simulink model "parallel_RFPSC_PSC_simulation"  (R2023b)
settings: Solver=VariableStepAuto  StartTime=0  StopTime=.1  FixedStep=T_s  MaxStep=T_s  RelTol=1e-4  AbsTol=1e-4  EnableMultiTasking=on
values from neighbouring files (symbols this model uses):
  f_sw = 10e3    (= 10000)    [init_psc_parallel.m]
  K_p = 3*w_g*R_a/(2*u_gN^2)    (= 0.261799387799)    [init_psc_parallel.m]
  L_f1 = L_f    (= 0.001)    [init_psc_parallel.m]
  L_f2 = L_f    (= 0.001)    [init_psc_parallel.m]
  L_g = 2.5e-3    (= 0.0025)    [init_psc_parallel.m]
  R_a = 0.32    [init_psc_parallel.m]
  R_L = 10    [init_psc_parallel.m]
  T_s = 1/(2*f_sw)    (= 5e-05)    [init_psc_parallel.m]
  U_dc = 48    [init_psc_parallel.m]
  u_gN = 24    [init_psc_parallel.m]
  w_g = 2*pi*50    (= 314.159265359)    [init_psc_parallel.m]    (also in psc_matlab.m = (P_ref - P)*K_p + w_1)
libraries: simulink x2
settings Model: Creator=mhinkkan  LastModifiedBy=jonwe
settings SolverCC: AutoScaleAbsTol=off  MaxConsecutiveMinStep=10  AlgebraicLoopSolver=TrustRegion
settings DataIOCC: SaveFormat=Array  SignalLoggingSaveFormat=ModelDataLogs  SaveOutput=off  SignalLogging=off  DSMLogging=off  SaveTime=off  ReturnWorkspaceOutputs=off
settings OptimizationCC: BlockReduction=off  BooleanDataType=off  DefaultParameterBehavior=Inlined  OptimizeBlockIOStorage=off  BufferReuse=off  ReuseModelBlockBuffer=off  ExpressionFolding=off  ExpressionDepthLimit=2147483647  LocalBlockOutputs=off  InitFltsAndDblsToZero=on  LifeSpan=inf
settings DebuggingCC: AlgebraicLoopMsg=none  SaveWithParameterizedLinksMsg=none  UnderspecifiedInitializationDetection=Classic  MergeDetectMultiDrivingBlocksExec=none  SignalResolutionControl=TryResolveAllWithWarning  MultiTaskDSMMsg=warning  MultiTaskCondExecSysMsg=none  FcnCallInpInsideContextMsg=warning  UnconnectedInputMsg=warning  UnconnectedOutputMsg=warning  UnconnectedLineMsg=warning  StateNameClashWarn=warning  SFUnexpectedBacktrackingDiag=warning  SFNoUnconditionalDefaultTransitionDiag=warning  SFExecutionAtInitializationDiag=none  ArithmeticOperatorsInVariantConditions=warning
settings HardwareCC: ProdBitPerPointer=32  ProdBitPerSizeT=32  ProdBitPerPtrDiffT=32  ProdLargestAtomicFloat=None  ProdIntDivRoundTo=Undefined  ProdEndianess=Unspecified  ProdWordSize=32  ProdHWDeviceType=32-bit Generic  TargetUnknown=on
settings ModelReferenceCC: PropagateSignalLabelsOutOfModel=off
settings SFSimCC: SimUseLocalCustomCode=off  CustomCodeUndefinedFunction=UseInterfaceOnly
settings RTWCC: RTWUseLocalCustomCode=off
settings CodeAppCC: StateflowObjectComments=on
settings GRTTargetCC: TargetFcnLib=ansi_tfl_tmw.mat  TargetLangStandard=C89/C90 (ANSI)  CombineOutputUpdateFcns=off  GRTInterface=on
settings ConfigComp: CovMetricSettings=dw  CovSaveCumulativeToWorkspaceVar=on  CovSaveSingleToWorkspaceVar=on  CovExternalEMLEnable=off

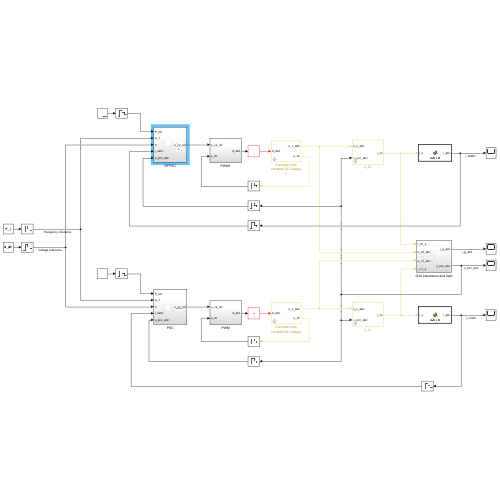
[thumbnail: Simulink's stored preview of the top-level diagram]
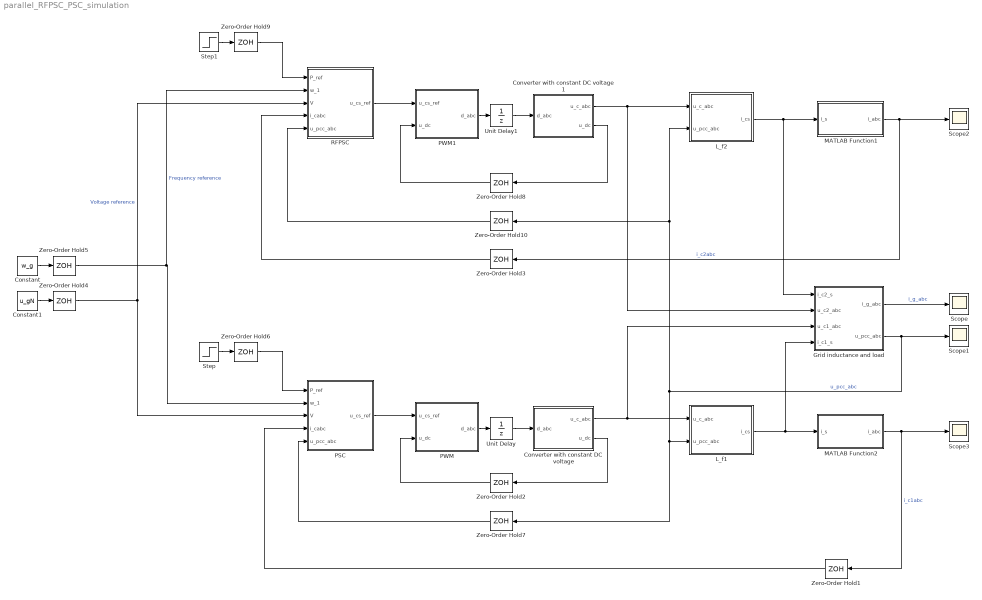
== system parallel_RFPSC_PSC_simulation ==
  Constant : Constant  Value=w_g
  Constant1 : Constant  Value=u_gN
  "Converter with constant DC voltage " : Subsystem  mask{f_sw=f_sw, u_dc=U_dc}
      mask prompts: f_sw "Switching frequency (Hz)"; u_dc "DC-bus voltage (V)"
      mask init:
      | T_s = 1/(2*f_sw);
  Converter with constant DC voltage 1 : Subsystem  mask{f_sw=f_sw, u_dc=U_dc}
      mask prompts: f_sw "Switching frequency (Hz)"; u_dc "DC-bus voltage (V)"
      mask init:
      | T_s = 1/(2*f_sw);
  Grid inductance and load : Subsystem
  L_f1 : Subsystem  mask{L_f=L_f1, R_f=0}
      mask prompts: L_f "Inductance (H)"; R_f "Series resistance (ohm)"
  L_f2 : Subsystem  mask{L_f=L_f2, R_f=0}
      mask prompts: L_f "Inductance (H)"; R_f "Series resistance (ohm)"
  MATLAB Function1 : MATLAB Function  TreatAsAtomicUnit=on
  MATLAB Function2 : MATLAB Function  TreatAsAtomicUnit=on
  PSC : Subsystem
  PWM : Subsystem
  PWM1 : Subsystem
  RFPSC : Subsystem
  Scope{,1..3} (4 alike) : Scope
  Step : Step  Time=.04  Before=10  After=20  SampleTime=T_s
  Step1 : Step  Time=.04  Before=20  After=10  SampleTime=T_s
  Unit Delay : UnitDelay  SampleTime=T_s  HasFrameUpgradeWarning=on
  Unit Delay1 : UnitDelay  SampleTime=T_s  HasFrameUpgradeWarning=on
  Zero-Order Hold{1..10} (10 alike) : ZeroOrderHold  SampleTime=T_s
  wires:
  L_f2/1(i_cs) -> Grid inductance and load/1(i_c2_s), MATLAB Function1/1(i_s)
  Grid inductance and load/1(i_g_abc) -> Scope/1  "i_g_abc"
  L_f1/1(i_cs) -> Grid inductance and load/4(i_c1_s), MATLAB Function2/1(i_s)
  MATLAB Function2/1(i_abc) -> Scope3/1, Zero-Order Hold1/1  "i_c1abc"
  Grid inductance and load/2(u_pcc_abc) -> Scope1/1, L_f2/2(u_pcc_abc), Zero-Order Hold10/1, Zero-Order Hold7/1, L_f1/2(u_pcc_abc)  "u_pcc_abc"
  "Converter with constant DC voltage "/2(u_dc) -> Zero-Order Hold2/1
  PWM/1(d_abc) -> Unit Delay/1
  Zero-Order Hold6/1 -> PSC/1(P_ref)
  Zero-Order Hold4/1 -> PSC/3(V), RFPSC/3(V)  "Voltage reference"
  Zero-Order Hold2/1 -> PWM/2(u_dc)
  Constant1/1 -> Zero-Order Hold4/1
  Step/1 -> Zero-Order Hold6/1
  Unit Delay/1 -> "Converter with constant DC voltage "/1(d_abc)
  Constant/1 -> Zero-Order Hold5/1
  Zero-Order Hold5/1 -> PSC/2(w_1), RFPSC/2(w_1)  "Frequency reference"
  Zero-Order Hold1/1 -> PSC/4(i_cabc)
  PSC/1(u_cs_ref) -> PWM/1(u_cs_ref)
  "Converter with constant DC voltage "/1(u_c_abc) -> Grid inductance and load/3(u_c1_abc), L_f1/1(u_c_abc)
  Zero-Order Hold7/1 -> PSC/5(u_pcc_abc)
  Zero-Order Hold10/1 -> RFPSC/5(u_pcc_abc)
  Converter with constant DC voltage 1/1(u_c_abc) -> L_f2/1(u_c_abc), Grid inductance and load/2(u_c2_abc)
  RFPSC/1(u_cs_ref) -> PWM1/1(u_cs_ref)
  Zero-Order Hold3/1 -> RFPSC/4(i_cabc)
  Unit Delay1/1 -> Converter with constant DC voltage 1/1(d_abc)
  Step1/1 -> Zero-Order Hold9/1
  Zero-Order Hold8/1 -> PWM1/2(u_dc)
  Zero-Order Hold9/1 -> RFPSC/1(P_ref)
  PWM1/1(d_abc) -> Unit Delay1/1
  Converter with constant DC voltage 1/2(u_dc) -> Zero-Order Hold8/1
  MATLAB Function1/1(i_abc) -> Zero-Order Hold3/1, Scope2/1  "i_c2abc"

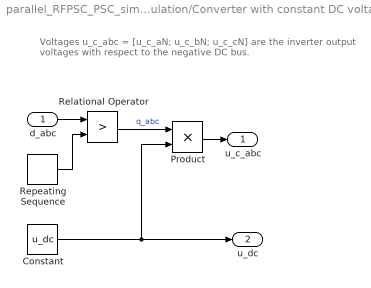
== system parallel_RFPSC_PSC_simulation/Converter with constant DC voltage  ==
  note: Voltages u_c_abc = [u_c_aN; u_c_bN; u_c_cN] are the inverter
      | output voltages with respect to the negative DC bus.
  d_abc : Inport
  Constant : Constant  Value=u_dc
  Product : Product
  Relational Operator : RelationalOperator  Operator=>  OutDataTypeStr='double'  InputSameDT=off
  Repeating Sequence : simulink/Sources/Repeating Sequence  rep_seq_t=[0 1 2]*T_s  rep_seq_y=[1 0 1]
  u_c_abc : Outport
  u_dc : Outport  Port=2
  wires:
  Repeating Sequence/1 -> Relational Operator/2
  d_abc/1 -> Relational Operator/1
  Product/1 -> u_c_abc/1
  Relational Operator/1 -> Product/1  "q_abc"
  Constant/1 -> Product/2, u_dc/1

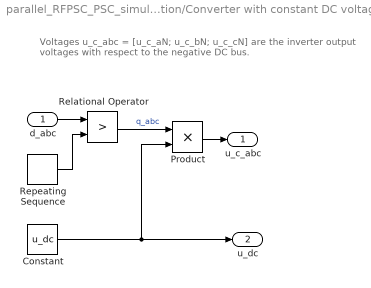
== system parallel_RFPSC_PSC_simulation/Converter with constant DC voltage 1 ==
  note: Voltages u_c_abc = [u_c_aN; u_c_bN; u_c_cN] are the inverter
      | output voltages with respect to the negative DC bus.
  d_abc : Inport
  Constant : Constant  Value=u_dc
  Product : Product
  Relational Operator : RelationalOperator  Operator=>  OutDataTypeStr='double'  InputSameDT=off
  Repeating Sequence : simulink/Sources/Repeating Sequence  rep_seq_t=[0 1 2]*T_s  rep_seq_y=[1 0 1]
  u_c_abc : Outport
  u_dc : Outport  Port=2
  wires:
  Constant/1 -> u_dc/1, Product/2
  Relational Operator/1 -> Product/1  "q_abc"
  Product/1 -> u_c_abc/1
  d_abc/1 -> Relational Operator/1
  Repeating Sequence/1 -> Relational Operator/2

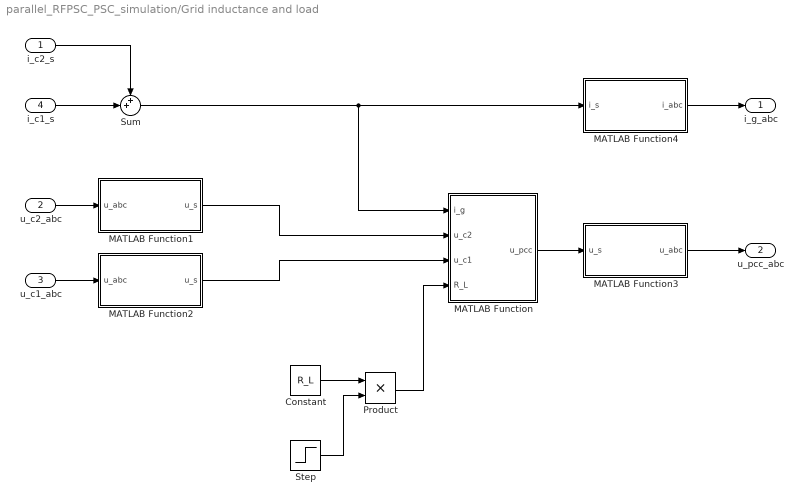
== system parallel_RFPSC_PSC_simulation/Grid inductance and load ==
  i_c2_s : Inport
  u_c2_abc : Inport  Port=2
  u_c1_abc : Inport  Port=3
  i_c1_s : Inport  Port=4
  Constant : Constant  Value=R_L
  MATLAB Function : MATLAB Function  TreatAsAtomicUnit=on
  MATLAB Function1 : MATLAB Function  TreatAsAtomicUnit=on
  MATLAB Function2 : MATLAB Function  TreatAsAtomicUnit=on
  MATLAB Function3 : MATLAB Function  TreatAsAtomicUnit=on
  MATLAB Function4 : MATLAB Function  TreatAsAtomicUnit=on
  Product : Product
  Step : Step  Time=.06  Before=1  After=0.5  SampleTime=0
  Sum : Sum  Inputs=++|
  i_g_abc : Outport
  u_pcc_abc : Outport  Port=2
  wires:
  Sum/1 -> MATLAB Function4/1(i_s), MATLAB Function/1(i_g)
  i_c2_s/1 -> Sum/1
  i_c1_s/1 -> Sum/2
  u_c2_abc/1 -> MATLAB Function1/1(u_abc)
  u_c1_abc/1 -> MATLAB Function2/1(u_abc)
  MATLAB Function1/1(u_s) -> MATLAB Function/2(u_c2)
  MATLAB Function2/1(u_s) -> MATLAB Function/3(u_c1)
  MATLAB Function/1(u_pcc) -> MATLAB Function3/1(u_s)
  MATLAB Function3/1(u_abc) -> u_pcc_abc/1
  MATLAB Function4/1(i_abc) -> i_g_abc/1
  Constant/1 -> Product/1
  Step/1 -> Product/2
  Product/1 -> MATLAB Function/4(R_L)

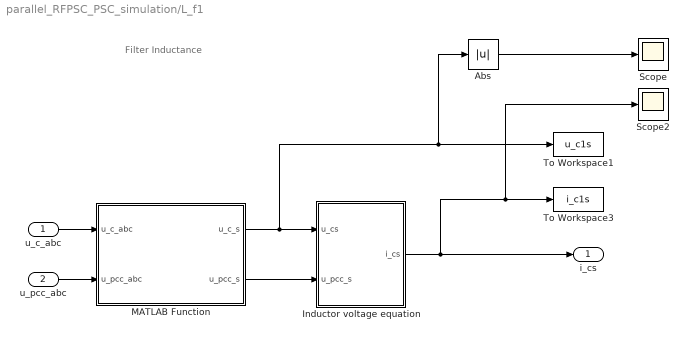
== system parallel_RFPSC_PSC_simulation/L_f1 ==
  note: Filter Inductance
  u_c_abc : Inport
  u_pcc_abc : Inport  Port=2
  Abs : Abs  SaturateOnIntegerOverflow=off
  Inductor voltage equation : Subsystem
  MATLAB Function : MATLAB Function  TreatAsAtomicUnit=on
  Scope : Scope
  Scope2 : Scope
  To Workspace1 : ToWorkspace  VariableName=u_c1s  SaveFormat=Timeseries
  To Workspace3 : ToWorkspace  VariableName=i_c1s  SaveFormat=Timeseries
  i_cs : Outport
  wires:
  Abs/1 -> Scope/1
  Inductor voltage equation/1(i_cs) -> i_cs/1, Scope2/1, To Workspace3/1
  MATLAB Function/1(u_c_s) -> Inductor voltage equation/1(u_cs), To Workspace1/1, Abs/1
  u_c_abc/1 -> MATLAB Function/1(u_c_abc)
  MATLAB Function/2(u_pcc_s) -> Inductor voltage equation/2(u_pcc_s)
  u_pcc_abc/1 -> MATLAB Function/2(u_pcc_abc)

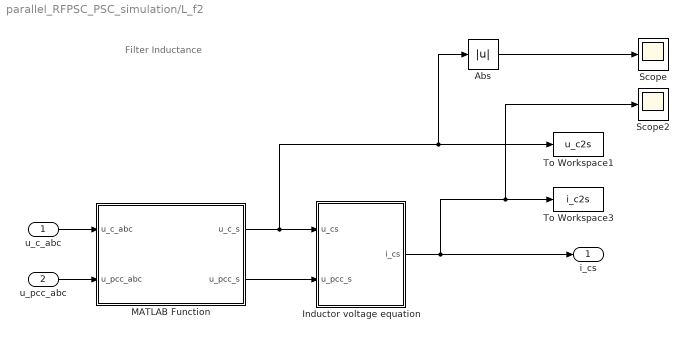
== system parallel_RFPSC_PSC_simulation/L_f2 ==
  note: Filter Inductance
  u_c_abc : Inport
  u_pcc_abc : Inport  Port=2
  Abs : Abs  SaturateOnIntegerOverflow=off
  Inductor voltage equation : Subsystem
  MATLAB Function : MATLAB Function  TreatAsAtomicUnit=on
  Scope : Scope
  Scope2 : Scope
  To Workspace1 : ToWorkspace  VariableName=u_c2s  SaveFormat=Timeseries
  To Workspace3 : ToWorkspace  VariableName=i_c2s  SaveFormat=Timeseries
  i_cs : Outport
  wires:
  Abs/1 -> Scope/1
  Inductor voltage equation/1(i_cs) -> i_cs/1, Scope2/1, To Workspace3/1
  MATLAB Function/1(u_c_s) -> Inductor voltage equation/1(u_cs), To Workspace1/1, Abs/1
  u_c_abc/1 -> MATLAB Function/1(u_c_abc)
  MATLAB Function/2(u_pcc_s) -> Inductor voltage equation/2(u_pcc_s)
  u_pcc_abc/1 -> MATLAB Function/2(u_pcc_abc)

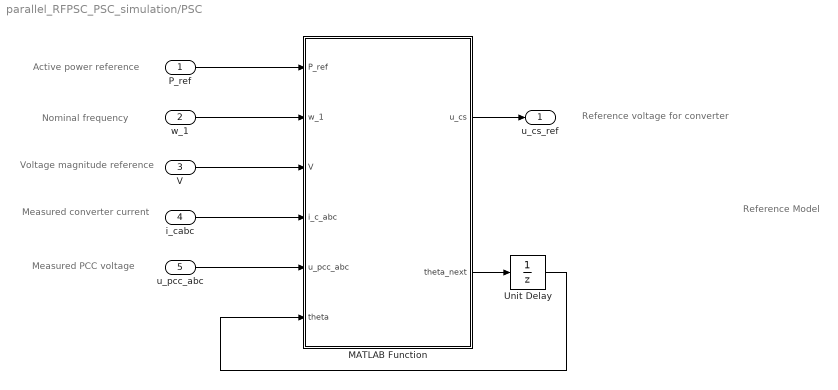
== system parallel_RFPSC_PSC_simulation/PSC ==
  note: Measured PCC voltage
  note: Voltage magnitude reference
  note: Nominal frequency
  note: Measured converter current
  note: Active power reference
  note: Reference voltage for converter
  note: Reference Model
  P_ref : Inport
  w_1 : Inport  Port=2
  V : Inport  Port=3
  i_cabc : Inport  Port=4
  u_pcc_abc : Inport  Port=5
  MATLAB Function : MATLAB Function  TreatAsAtomicUnit=on
  Unit Delay : UnitDelay  SampleTime=-1  HasFrameUpgradeWarning=on
  u_cs_ref : Outport
  wires:
  MATLAB Function/2(theta_next) -> Unit Delay/1
  Unit Delay/1 -> MATLAB Function/6(theta)
  P_ref/1 -> MATLAB Function/1(P_ref)
  w_1/1 -> MATLAB Function/2(w_1)
  V/1 -> MATLAB Function/3(V)
  u_pcc_abc/1 -> MATLAB Function/5(u_pcc_abc)
  i_cabc/1 -> MATLAB Function/4(i_c_abc)
  MATLAB Function/1(u_cs) -> u_cs_ref/1

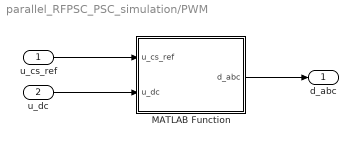
== system parallel_RFPSC_PSC_simulation/PWM ==
  u_cs_ref : Inport
  u_dc : Inport  Port=2
  MATLAB Function : MATLAB Function  TreatAsAtomicUnit=on
  d_abc : Outport
  wires:
  u_cs_ref/1 -> MATLAB Function/1(u_cs_ref)
  MATLAB Function/1(d_abc) -> d_abc/1
  u_dc/1 -> MATLAB Function/2(u_dc)

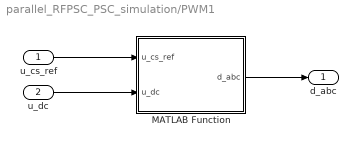
== system parallel_RFPSC_PSC_simulation/PWM1 ==
  u_cs_ref : Inport
  u_dc : Inport  Port=2
  MATLAB Function : MATLAB Function  TreatAsAtomicUnit=on
  d_abc : Outport
  wires:
  u_dc/1 -> MATLAB Function/2(u_dc)
  MATLAB Function/1(d_abc) -> d_abc/1
  u_cs_ref/1 -> MATLAB Function/1(u_cs_ref)

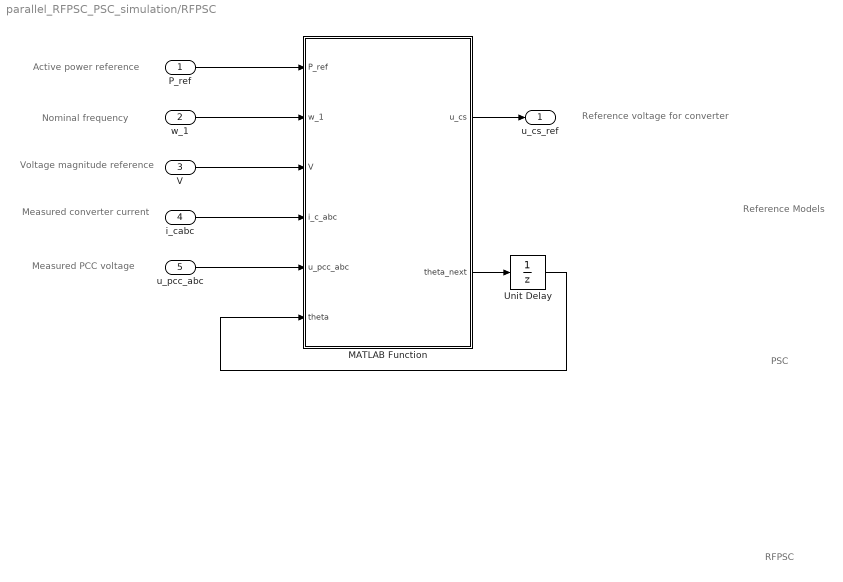
== system parallel_RFPSC_PSC_simulation/RFPSC ==
  note: RFPSC
  note: Measured PCC voltage
  note: Voltage magnitude reference
  note: Nominal frequency
  note: Measured converter current
  note: Active power reference
  note: Reference voltage for converter
  note: Reference Models
  note: PSC
  P_ref : Inport
  w_1 : Inport  Port=2
  V : Inport  Port=3
  i_cabc : Inport  Port=4
  u_pcc_abc : Inport  Port=5
  MATLAB Function : MATLAB Function  TreatAsAtomicUnit=on
  Unit Delay : UnitDelay  SampleTime=-1  HasFrameUpgradeWarning=on
  u_cs_ref : Outport
  wires:
  MATLAB Function/2(theta_next) -> Unit Delay/1
  Unit Delay/1 -> MATLAB Function/6(theta)
  P_ref/1 -> MATLAB Function/1(P_ref)
  w_1/1 -> MATLAB Function/2(w_1)
  V/1 -> MATLAB Function/3(V)
  u_pcc_abc/1 -> MATLAB Function/5(u_pcc_abc)
  i_cabc/1 -> MATLAB Function/4(i_c_abc)
  MATLAB Function/1(u_cs) -> u_cs_ref/1

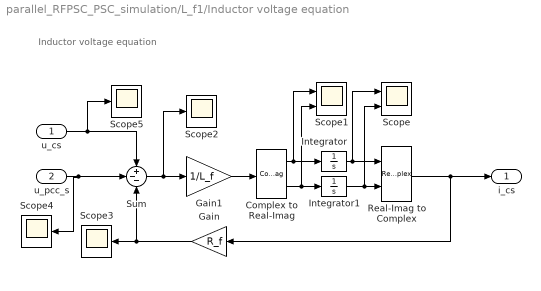
== system parallel_RFPSC_PSC_simulation/L_f1/Inductor voltage equation ==
  note: Inductor voltage equation
  u_cs : Inport
  u_pcc_s : Inport  Port=2
  Complex to Real-Imag : ComplexToRealImag
  Gain : Gain  Gain=R_f
  Gain1 : Gain  Gain=1/L_f
  Integrator : Integrator
  Integrator1 : Integrator
  Real-Imag to Complex : RealImagToComplex
  Scope : Scope  NumInputPorts=2
  Scope1 : Scope  NumInputPorts=2
  Scope{2..5} (4 alike) : Scope
  Sum : Sum  Inputs=+--
  i_cs : Outport
  wires:
  Gain/1 -> Scope3/1, Sum/3
  Real-Imag to Complex/1 -> i_cs/1, Gain/1
  Integrator1/1 -> Real-Imag to Complex/2, Scope/2
  Integrator/1 -> Real-Imag to Complex/1, Scope/1
  Complex to Real-Imag/2 -> Integrator1/1, Scope1/2
  Complex to Real-Imag/1 -> Integrator/1, Scope1/1
  Gain1/1 -> Complex to Real-Imag/1
  Sum/1 -> Scope2/1, Gain1/1
  u_pcc_s/1 -> Scope4/1, Sum/2
  u_cs/1 -> Scope5/1, Sum/1

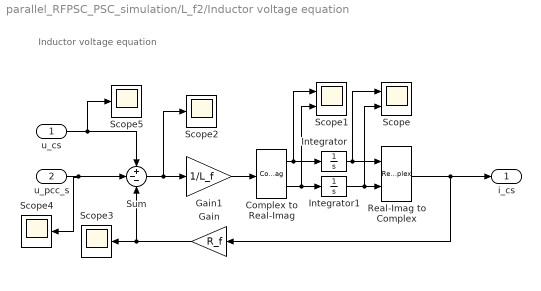
== system parallel_RFPSC_PSC_simulation/L_f2/Inductor voltage equation ==
  note: Inductor voltage equation
  u_cs : Inport
  u_pcc_s : Inport  Port=2
  Complex to Real-Imag : ComplexToRealImag
  Gain : Gain  Gain=R_f
  Gain1 : Gain  Gain=1/L_f
  Integrator : Integrator
  Integrator1 : Integrator
  Real-Imag to Complex : RealImagToComplex
  Scope : Scope  NumInputPorts=2
  Scope1 : Scope  NumInputPorts=2
  Scope{2..5} (4 alike) : Scope
  Sum : Sum  Inputs=+--
  i_cs : Outport
  wires:
  Gain/1 -> Scope3/1, Sum/3
  Real-Imag to Complex/1 -> i_cs/1, Gain/1
  Integrator1/1 -> Real-Imag to Complex/2, Scope/2
  Integrator/1 -> Real-Imag to Complex/1, Scope/1
  Complex to Real-Imag/2 -> Integrator1/1, Scope1/2
  Complex to Real-Imag/1 -> Integrator/1, Scope1/1
  Gain1/1 -> Complex to Real-Imag/1
  Sum/1 -> Scope2/1, Gain1/1
  u_pcc_s/1 -> Scope4/1, Sum/2
  u_cs/1 -> Scope5/1, Sum/1

== matlab function parallel_RFPSC_PSC_simulation/Grid inductance and load/MATLAB Function1 ==
  data: u_abc input size=3; u_s output size=1
function u_s = abc2s(u_abc)

% Space-vector transformation
u_s = 2/3*(u_abc(1) + u_abc(2)*exp(1j*2*pi/3) + u_abc(3)*exp(1j*4*pi/3));

== matlab function parallel_RFPSC_PSC_simulation/Grid inductance and load/MATLAB Function2 ==
  data: u_abc input size=3; u_s output size=1
function u_s = abc2s(u_abc)

% Space-vector transformation
u_s = 2/3*(u_abc(1) + u_abc(2)*exp(1j*2*pi/3) + u_abc(3)*exp(1j*4*pi/3));

== matlab function parallel_RFPSC_PSC_simulation/Grid inductance and load/MATLAB Function3 ==
  data: u_s input size=1; u_abc output size=3
function u_abc = s2abc(u_s)

% Inverse space-vector transformation
u_abc = real([1; exp(-1j*2*pi/3); exp(-1j*4*pi/3)]*u_s);

== matlab function parallel_RFPSC_PSC_simulation/Grid inductance and load/MATLAB Function4 ==
  data: i_s input size=1; i_abc output size=3
function i_abc = s2abc(i_s)

% Inverse space-vector transformation
i_abc = real([1; exp(-1j*2*pi/3); exp(-1j*4*pi/3)]*i_s);

== matlab function parallel_RFPSC_PSC_simulation/L_f1/MATLAB Function ==
  data: u_c_abc input; u_pcc_abc input; u_c_s output; u_pcc_s output
function [u_c_s, u_pcc_s] = abc2s(u_c_abc, u_pcc_abc)

% Space Vector Transformation of converter and pcc voltage
u_c_s = 2/3*(u_c_abc(1) + u_c_abc(2)*exp(1j*2*pi/3) + u_c_abc(3)*exp(1j*4*pi/3));

u_pcc_s = 2/3*(u_pcc_abc(1) + u_pcc_abc(2)*exp(1j*2*pi/3) + u_pcc_abc(3)*exp(1j*4*pi/3));

== matlab function parallel_RFPSC_PSC_simulation/PSC/MATLAB Function ==
  data: P_ref input; u_cs output; theta_next output; w_1 input; V input; i_c_abc input; u_pcc_abc input; theta input; K_p parameter; T_s parameter; R_a parameter
function [u_cs, theta_next] = PSC(P_ref, w_1, V, i_c_abc, u_pcc_abc, ...
    theta, K_p, T_s, R_a)

% Space Vector Transformation of PCC voltage (abcTos)
u_pcc_s = 2/3*(u_pcc_abc(1) + u_pcc_abc(2)*exp(1j*2*pi/3) + u_pcc_abc(3)*exp(1j*4*pi/3));

% Space Vector Transformation of converter current (abcTos)
i_cs = 2/3*(i_c_abc(1) + i_c_abc(2)*exp(1j*2*pi/3) + i_c_abc(3)*exp(1j*4*pi/3));

% Active power calculation
P = 3/2*real(u_pcc_s*conj(i_cs));

% Equation for grid angular frequency
w_g = (P_ref - P)*K_p + w_1;

% Update (integrate) the grid voltage angle
theta_next = theta + T_s * w_g;

% Coordinate transformation of converter current
i_c = i_cs*exp(-1j*theta_next);

% Extracting the real and imaginary values of the complex converter current
i_c_real = real(i_c);
i_c_imag = imag(i_c);

% Applying highpass filter equation to real and imaginary parts of the
% converter current
i_c_filtered_real =  i_c_real - i_c_real/T_s * exp(-1/T_s);
i_c_filtered_imag =  i_c_imag - i_c_imag/T_s * exp(-1/T_s);

% Equation for reference voltage
u_c = V - (i_c_filtered_real + 1j*i_c_filtered_imag) * R_a;

% Inverse coordinate transformation
u_cs = u_c*exp(1j*theta_next);

== matlab function parallel_RFPSC_PSC_simulation/PWM/MATLAB Function ==
  data: d_abc output; u_cs_ref input; u_dc input
function d_abc = fcn(u_cs_ref, u_dc)

%% Symmetrical suboscillation PWM
% Components of the voltage space vector
u_c_alpha_ref = real(u_cs_ref);
u_c_beta_ref  = imag(u_cs_ref);

% Phase-voltage references
u_ca_ref = u_c_alpha_ref;
u_cb_ref = .5*(-u_c_alpha_ref + sqrt(3)*u_c_beta_ref);
u_cc_ref = .5*(-u_c_alpha_ref - sqrt(3)*u_c_beta_ref);

% Vector of phase-voltage references
u_c_abc_ref = [u_ca_ref; u_cb_ref; u_cc_ref];

% Symmetrization of the references by adding the zero-sequence voltage
u0 = .5*(max(u_c_abc_ref) + min(u_c_abc_ref));
u_c_abc_ref = u_c_abc_ref - u0;

% Clipping of the reference voltages such that no phase error is caused. 
% If all phase voltage reference are realizable (below u_dc/2), m = 1 holds.
m = max([2*u_c_abc_ref/u_dc; 1]);
u_c_abc_ref = u_c_abc_ref/m;

% Duty cycles, which can be directly used for triangle comparison, 
% if the triangle wave varies between 0...1
d_abc = .5 + u_c_abc_ref/u_dc;
% 
% % Realized voltage vector is calculated from the clamped duty ratios.
% % If the PWM does not saturate, u_c_ref_lim = u_c_ref holds. The realized
% % voltage vector is needed, e.g., for the current-controller antiwindup.
% u_cs_ref_lim = 2/3*(d_abc(1) + d_abc(2)*exp(1j*2*pi/3) ...
%     + d_abc(3)*exp(1j*4*pi/3))*u_dc;
% % In estimated rotor flux coordinates
% u_c_ref_lim = exp(-1j*theta)*u_cs_ref_lim;

== matlab function parallel_RFPSC_PSC_simulation/L_f2/MATLAB Function ==
  data: u_c_abc input; u_pcc_abc input; u_c_s output; u_pcc_s output
function [u_c_s, u_pcc_s] = abc2s(u_c_abc, u_pcc_abc)

% Space Vector Transformation of converter and pcc voltage
u_c_s = 2/3*(u_c_abc(1) + u_c_abc(2)*exp(1j*2*pi/3) + u_c_abc(3)*exp(1j*4*pi/3));

u_pcc_s = 2/3*(u_pcc_abc(1) + u_pcc_abc(2)*exp(1j*2*pi/3) + u_pcc_abc(3)*exp(1j*4*pi/3));

== matlab function parallel_RFPSC_PSC_simulation/RFPSC/MATLAB Function ==
  data: P_ref input; u_cs output; theta_next output; w_1 input; V input; i_c_abc input; u_pcc_abc input; theta input; K_p parameter; T_s parameter; R_a parameter
function [u_cs, theta_next] = RFPSC(P_ref, w_1, V, i_c_abc, u_pcc_abc, ...
    theta, K_p, T_s, R_a)

% Space Vector Transformation of PCC voltage (abcTos)
u_pcc_s = 2/3*(u_pcc_abc(1) + u_pcc_abc(2)*exp(1j*2*pi/3) + u_pcc_abc(3)*exp(1j*4*pi/3));

% Space Vector Transformation of converter current (abcTos)
i_cs = 2/3*(i_c_abc(1) + i_c_abc(2)*exp(1j*2*pi/3) + i_c_abc(3)*exp(1j*4*pi/3));

% Active power calculation
P = 3/2*real(u_pcc_s*conj(i_cs));

% Equation for grid angular frequency
w_g = (P_ref - P)*K_p + w_1;

% Update (integrate) the grid voltage angle
theta_next = theta + T_s * w_g;

% Coordinate transformation of converter current
i_c = i_cs*exp(-1j*theta_next);

% Extracting the real and imaginary values of the complex converter current
i_c_imag = imag(i_c);

% Applying highpass filter equation to imaginary part of the
% converter current and forming reference current based on power reference
i_c_filtered_imag =  i_c_imag - i_c_imag/T_s * exp(-1/T_s);
i_ref = P_ref/V + 1j*i_c_filtered_imag;

% Equation for reference voltage
u_c = V + (i_ref-i_c) * R_a;

% Inverse coordinate transformation
u_cs = u_c*exp(1j*theta_next);

== matlab function parallel_RFPSC_PSC_simulation/MATLAB Function1 ==
  data: i_s input size=1; i_abc output size=3
function i_abc = s2abc(i_s)

% Inverse space-vector transformation
i_abc = real([1; exp(-1j*2*pi/3); exp(-1j*4*pi/3)]*i_s);

== matlab function parallel_RFPSC_PSC_simulation/MATLAB Function2 ==
  data: i_s input size=1; i_abc output size=3
function i_abc = s2abc(i_s)

% Inverse space-vector transformation
i_abc = real([1; exp(-1j*2*pi/3); exp(-1j*4*pi/3)]*i_s);

== matlab function parallel_RFPSC_PSC_simulation/PWM1/MATLAB Function ==
  data: d_abc output; u_cs_ref input; u_dc input
function d_abc = fcn(u_cs_ref, u_dc)

%% Symmetrical suboscillation PWM
% Components of the voltage space vector
u_c_alpha_ref = real(u_cs_ref);
u_c_beta_ref  = imag(u_cs_ref);

% Phase-voltage references
u_ca_ref = u_c_alpha_ref;
u_cb_ref = .5*(-u_c_alpha_ref + sqrt(3)*u_c_beta_ref);
u_cc_ref = .5*(-u_c_alpha_ref - sqrt(3)*u_c_beta_ref);

% Vector of phase-voltage references
u_c_abc_ref = [u_ca_ref; u_cb_ref; u_cc_ref];

% Symmetrization of the references by adding the zero-sequence voltage
u0 = .5*(max(u_c_abc_ref) + min(u_c_abc_ref));
u_c_abc_ref = u_c_abc_ref - u0;

% Clipping of the reference voltages such that no phase error is caused. 
% If all phase voltage reference are realizable (below u_dc/2), m = 1 holds.
m = max([2*u_c_abc_ref/u_dc; 1]);
u_c_abc_ref = u_c_abc_ref/m;

% Duty cycles, which can be directly used for triangle comparison, 
% if the triangle wave varies between 0...1
d_abc = .5 + u_c_abc_ref/u_dc;
% 
% % Realized voltage vector is calculated from the clamped duty ratios.
% % If the PWM does not saturate, u_c_ref_lim = u_c_ref holds. The realized
% % voltage vector is needed, e.g., for the current-controller antiwindup.
% u_cs_ref_lim = 2/3*(d_abc(1) + d_abc(2)*exp(1j*2*pi/3) ...
%     + d_abc(3)*exp(1j*4*pi/3))*u_dc;
% % In estimated rotor flux coordinates
% u_c_ref_lim = exp(-1j*theta)*u_cs_ref_lim;

== matlab function parallel_RFPSC_PSC_simulation/Grid inductance and load/MATLAB Function ==
  data: i_g input; u_pcc output; u_c2 input; L_g parameter; L_f1 parameter; L_f2 parameter; u_c1 input; R_L input
function u_pcc = fcn(i_g, u_c2, L_g, L_f1, L_f2, u_c1, R_L)

u_pcc = (L_g*(u_c1/L_f1+u_c2/L_f2)+R_L*i_g)/(1+L_g/L_f1+L_g/L_f2);
